simulink model "lat747mod9"  (Simulink 8.2)
settings: Solver=ode45  StartTime=0.0  StopTime=200  RelTol=1e-8  AbsTol=1e-8
values from neighbouring files (symbols this model uses):
  B = B(:,1:2)    [TwoTankSystem.m]
  K = K_of(:,1:4)    [TwoTankSystem.m]
undefined symbols (not defined in the file or in its folder): A, C
settings Model: Creator=OJ  LastModifiedBy=soene  ExtModeTrigMode=oneshot  ExtModeArmWhenConnect=off
settings DataIOCC: LimitDataPoints=off  SaveOutput=off
settings OptimizationCC: BooleanDataType=off  InitFltsAndDblsToZero=on
settings DebuggingCC: SaveWithParameterizedLinksMsg=none  SignalResolutionControl=TryResolveAllWithWarning  SolverPrmCheckMsg=none  MultiTaskDSMMsg=warning  MultiTaskCondExecSysMsg=none  UnconnectedInputMsg=none  UnconnectedOutputMsg=none  StrictBusMsg=None
settings HardwareCC: TargetUnknown=on
settings RTWCC: IncludeERTFirstTime=on
settings CodeAppCC: IgnoreCustomStorageClasses=off
settings GRTTargetCC: TargetFcnLib=ansi_tfl_tmw.mat

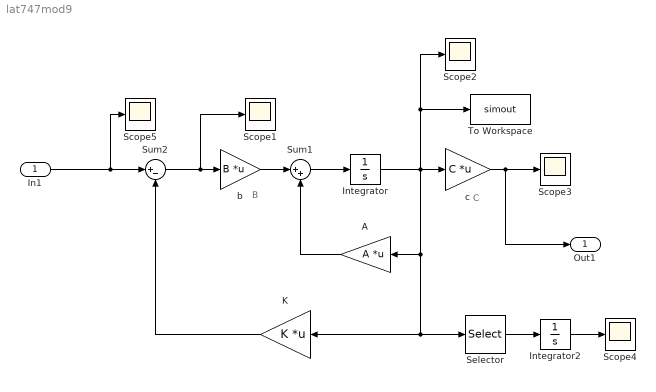
== system lat747mod9 ==
  note: B
  note: C
  In1 : Inport  PortDimensions=2
  A : Gain  Gain=A  Multiplication=Matrix(K*u)  SaturateOnIntegerOverflow=on  OutDataTypeStr=Inherit: Same as input  ParamDataTypeStr=Inherit: Same as input
  Integrator : Integrator  InitialCondition=0%[.0175 0 0 0]'
  Integrator2 : Integrator  InitialCondition=0%[.0175 0 0 0]'
  K : Gain  Gain=K  Multiplication=Matrix(K*u)  SaturateOnIntegerOverflow=on  OutDataTypeStr=Inherit: Same as input  ParamDataTypeStr=Inherit: Same as input
  Scope{1..5} (5 alike) : Scope
      Scope3 settings: SaveName=ScopeData2
      Scope4 settings: SaveName=ScopeData3
      Scope5 settings: SaveName=ScopeData4
  Selector : Selector  InputPortWidth=4  IndexOptions=Index vector (dialog)  Indices=[2]  OutputSizes=1
  Sum1 : Sum  Inputs=|++  SaturateOnIntegerOverflow=on  InputSameDT=on  OutDataTypeStr=Inherit: Same as first input
  Sum2 : Sum  Inputs=|+-  SaturateOnIntegerOverflow=on  InputSameDT=on  OutDataTypeStr=Inherit: Same as first input
  To Workspace : ToWorkspace  VariableName=simout  SampleTime=-1
  b : Gain  Gain=B  Multiplication=Matrix(K*u)  SaturateOnIntegerOverflow=on  OutDataTypeStr=Inherit: Same as input  ParamDataTypeStr=Inherit: Same as input
  c : Gain  Gain=C  Multiplication=Matrix(K*u)  SaturateOnIntegerOverflow=on  OutDataTypeStr=Inherit: Same as input  ParamDataTypeStr=Inherit: Same as input
  Out1 : Outport
  wires:
  Integrator/1 -> Scope2/1, To Workspace/1, c/1, A/1, K/1, Selector/1
  Sum1/1 -> Integrator/1
  b/1 -> Sum1/1
  A/1 -> Sum1/2
  c/1 -> Scope3/1, Out1/1
  Sum2/1 -> b/1, Scope1/1
  In1/1 -> Sum2/1, Scope5/1
  Selector/1 -> Integrator2/1
  Integrator2/1 -> Scope4/1
  K/1 -> Sum2/2
